simulink model "f_cd_reorder_one_interface"  (R2018a)
settings: Solver=VariableStepAuto  StartTime=0.0  StopTime=200000  RelTol=1e-3
libraries: xbsIndex_r4 x1754, casper_library_misc x12, xps_library x2, simulink x1
(part 2 of 9)

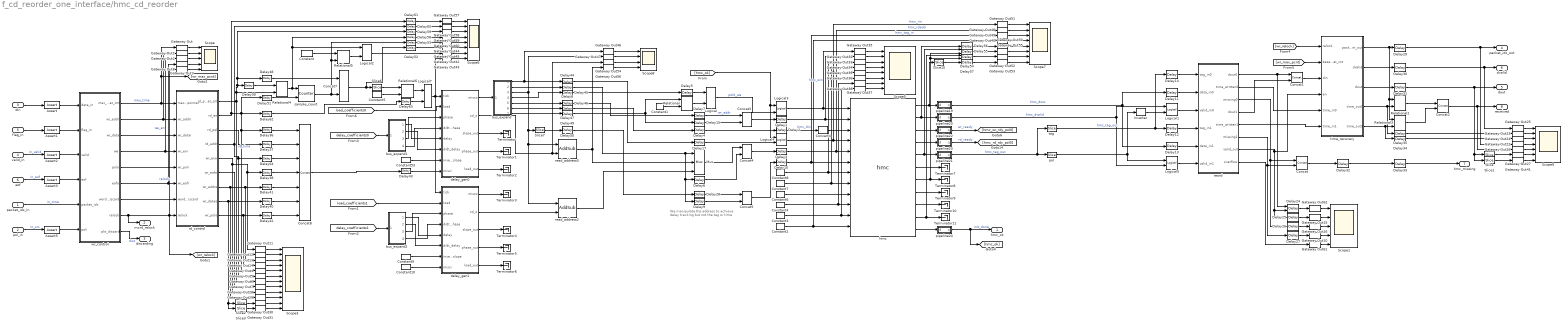
== system f_cd_reorder_one_interface/hmc_cd_reorder ==
  note: We manipulate the address to
      | achieve delay tracking but not the tag
      | or time
  packet_idx_in : Inport
  pol_in : Inport  Port=2
  din : Inport  Port=3
  valid_in : Inport  Port=4
  flag_in : Inport  Port=5
  eof : Inport  Port=6
  Assert : xbsIndex_r4/Assert  assert_type=on  type_source=Explicitly  gui_display_data_type=Fixed-point  arith_type=Unsigned  n_bits=n_bits_din  bin_pt=0  preci_type=Single  exp_width=8  frac_width=24  assert_rate=off  rate_source=Explicitly  period=1  output_port=on  block_type=assert
  Assert1 : xbsIndex_r4/Assert  assert_type=on  type_source=Explicitly  gui_display_data_type=Fixed-point  arith_type=Unsigned  n_bits=n_bits_flag  bin_pt=0  preci_type=Single  exp_width=8  frac_width=24  assert_rate=off  rate_source=Explicitly  period=1  output_port=on  block_type=assert
  Assert2 : xbsIndex_r4/Assert  assert_type=on  type_source=Explicitly  gui_display_data_type=Boolean  arith_type=Boolean  n_bits=n_bits_flag  bin_pt=0  preci_type=Single  exp_width=8  frac_width=24  assert_rate=off  rate_source=Explicitly  period=1  output_port=on  block_type=assert
  Assert3 : xbsIndex_r4/Assert  assert_type=on  type_source=Explicitly  gui_display_data_type=Boolean  arith_type=Boolean  n_bits=n_bits_flag  bin_pt=0  preci_type=Single  exp_width=8  frac_width=24  assert_rate=off  rate_source=Explicitly  period=1  output_port=on  block_type=assert
  Assert5 : xbsIndex_r4/Assert  assert_type=on  type_source=Explicitly  gui_display_data_type=Fixed-point  arith_type=Unsigned  n_bits=1  bin_pt=0  preci_type=Single  exp_width=8  frac_width=24  assert_rate=off  rate_source=Explicitly  period=1  output_port=on  block_type=assert
  Concat{,1..5,7} (7 alike) : xbsIndex_r4/Concat  num_inputs=2  dbl_ovrd=off  block_type=concat
  Concat8 : xbsIndex_r4/Concat  num_inputs=7  dbl_ovrd=off  block_type=concat
  Constant : xbsIndex_r4/Constant  const=(packet_size-1)*samples_per_word*2  gui_display_data_type=Fixed-point  arith_type=Unsigned  n_bits=ceil(log2(packet_size*samples_per_word))+1  bin_pt=0  preci_type=Single  exp_width=8  frac_width=24  explicit_period=on  period=1  equ=P=C  opselect=C  inp2=PCIN>>17  opr=+  inp1=P  carry=CIN  dbl_ovrd=off  block_type=constant
  Constant1 : xbsIndex_r4/Constant  const=0  gui_display_data_type=Fixed-point  arith_type=Unsigned  n_bits=1  bin_pt=0  preci_type=Single  exp_width=8  frac_width=24  explicit_period=on  period=1  equ=P=C  opselect=C  inp2=PCIN>>17  opr=+  inp1=P  carry=CIN  dbl_ovrd=off  block_type=constant
  Constant10 : xbsIndex_r4/Constant  const=0  gui_display_data_type=Boolean  arith_type=Boolean  n_bits=1  bin_pt=0  preci_type=Single  exp_width=8  frac_width=24  explicit_period=on  period=1  equ=P=C  opselect=C  inp2=PCIN>>17  opr=+  inp1=P  carry=CIN  dbl_ovrd=off  block_type=constant
      settings: block_version=11.4
  Constant2 : xbsIndex_r4/Constant  const=0  gui_display_data_type=Fixed-point  arith_type=Unsigned  n_bits=9  bin_pt=0  preci_type=Single  exp_width=8  frac_width=24  explicit_period=on  period=1  equ=P=C  opselect=C  inp2=PCIN>>17  opr=+  inp1=P  carry=CIN  dbl_ovrd=off  block_type=constant
  Constant3 : xbsIndex_r4/Constant  const=0  gui_display_data_type=Fixed-point  arith_type=Unsigned  n_bits=n_bits_buffer_size  bin_pt=0  preci_type=Single  exp_width=8  frac_width=24  explicit_period=on  period=1  equ=P=C  opselect=C  inp2=PCIN>>17  opr=+  inp1=P  carry=CIN  dbl_ovrd=off  block_type=constant
  Constant4 : xbsIndex_r4/Constant  const=0  gui_display_data_type=Boolean  arith_type=Boolean  n_bits=n_bits_buffer_size  bin_pt=0  preci_type=Single  exp_width=8  frac_width=24  explicit_period=on  period=1  equ=P=C  opselect=C  inp2=PCIN>>17  opr=+  inp1=P  carry=CIN  dbl_ovrd=off  block_type=constant
  Constant5 : xbsIndex_r4/Constant  const=0  gui_display_data_type=Fixed-point  arith_type=Unsigned  n_bits=n_bits_fft+1  bin_pt=0  preci_type=Single  exp_width=8  frac_width=24  explicit_period=on  period=1  equ=P=C  opselect=C  inp2=PCIN>>17  opr=+  inp1=P  carry=CIN  dbl_ovrd=off  block_type=constant
  Constant53 : xbsIndex_r4/Constant  const=0  gui_display_data_type=Boolean  arith_type=Boolean  n_bits=1  bin_pt=0  preci_type=Single  exp_width=8  frac_width=24  explicit_period=on  period=1  equ=P=C  opselect=C  inp2=PCIN>>17  opr=+  inp1=P  carry=CIN  dbl_ovrd=off  block_type=constant
      settings: block_version=11.4
  Constant6 : xbsIndex_r4/Constant  const=0  gui_display_data_type=Fixed-point  arith_type=Unsigned  n_bits=256  bin_pt=0  preci_type=Single  exp_width=8  frac_width=24  explicit_period=on  period=1  equ=P=C  opselect=C  inp2=PCIN>>17  opr=+  inp1=P  carry=CIN  dbl_ovrd=off  block_type=constant
  Constant7 : xbsIndex_r4/Constant  const=0  gui_display_data_type=Fixed-point  arith_type=Unsigned  n_bits=n_bits_buffer_size  bin_pt=0  preci_type=Single  exp_width=8  frac_width=24  explicit_period=on  period=1  equ=P=C  opselect=C  inp2=PCIN>>17  opr=+  inp1=P  carry=CIN  dbl_ovrd=off  block_type=constant
  Constant8 : xbsIndex_r4/Constant  const=0  gui_display_data_type=Boolean  arith_type=Boolean  n_bits=n_bits_buffer_size  bin_pt=0  preci_type=Single  exp_width=8  frac_width=24  explicit_period=on  period=1  equ=P=C  opselect=C  inp2=PCIN>>17  opr=+  inp1=P  carry=CIN  dbl_ovrd=off  block_type=constant
  Constant9 : xbsIndex_r4/Constant  const=0  gui_display_data_type=Boolean  arith_type=Boolean  n_bits=1  bin_pt=0  preci_type=Single  exp_width=8  frac_width=24  explicit_period=on  period=1  equ=P=C  opselect=C  inp2=PCIN>>17  opr=+  inp1=P  carry=CIN  dbl_ovrd=off  block_type=constant
      settings: block_version=11.4
  Convert4 : xbsIndex_r4/Convert  gui_display_data_type=Fixed-point  arith_type=Unsigned  n_bits=256  bin_pt=0  float_type=Single  exp_bits=8  fraction_bits=24  quantization=Truncate  overflow=Wrap  en=off  latency=0  pipeline=off  dbl_ovrd=off  block_type=convert
  Delay{1..3,5,8,10..14,43..53,56..63} (29 alike) : xbsIndex_r4/Delay  rst=off  infoeditControl=Selection of Reset will increase slice count due to use of real FFs and instead of SRLs  en=off  latency=1  reg_retiming=on  dbl_ovrd=off  block_type=delay
      Delay1 settings: xl_area=[0, 0, 0, 0, 0, 0, 0]
      Delay10 settings: xl_area=[0, 0, 0, 0, 0, 0, 0]
      Delay2 settings: xl_area=[0, 0, 0, 0, 0, 0, 0]
      Delay3 settings: xl_area=[0, 0, 0, 0, 0, 0, 0]
      Delay44 settings: xl_area=[0, 0, 0, 0, 0, 0, 0]
      Delay45 settings: xl_area=[0, 0, 0, 0, 0, 0, 0]
      Delay46 settings: xl_area=[0, 0, 0, 0, 0, 0, 0]
      Delay47 settings: xl_area=[0, 0, 0, 0, 0, 0, 0]
      Delay49 settings: xl_area=[0, 0, 0, 0, 0, 0, 0]
      Delay5 settings: xl_area=[0, 0, 0, 0, 0, 0, 0]
      Delay50 settings: xl_area=[0, 0, 0, 0, 0, 0, 0]
      Delay56 settings: xl_area=[0, 0, 0, 0, 0, 0, 0]
      Delay57 settings: xl_area=[0, 0, 0, 0, 0, 0, 0]
      Delay8 settings: xl_area=[0, 0, 0, 0, 0, 0, 0]
  Delay{4,6..7,9,15,17,28} (7 alike) : xbsIndex_r4/Delay  rst=off  infoeditControl=Selection of Reset will increase slice count due to use of real FFs and instead of SRLs  en=off  latency=2  reg_retiming=on  dbl_ovrd=off  block_type=delay
      settings: xl_area=[0, 0, 0, 0, 0, 0, 0]
  Delay24 : xbsIndex_r4/Delay  rst=off  infoeditControl=Selection of Reset will increase slice count due to use of real FFs and instead of SRLs  en=on  latency=1  reg_retiming=off  dbl_ovrd=off  block_type=delay
  Delay{25..27,29..31,33..42,64} (17 alike) : xbsIndex_r4/Delay  rst=off  infoeditControl=Selection of Reset will increase slice count due to use of real FFs and instead of SRLs  en=off  latency=1  reg_retiming=off  dbl_ovrd=off  block_type=delay
  Delay32 : xbsIndex_r4/Delay  rst=off  infoeditControl=Selection of Reset will increase slice count due to use of real FFs and instead of SRLs  en=off  latency=2  reg_retiming=off  dbl_ovrd=off  block_type=delay
  Delay54 : xbsIndex_r4/Delay  rst=off  infoeditControl=Selection of Reset will increase slice count due to use of real FFs and instead of SRLs  en=on  latency=1  reg_retiming=on  dbl_ovrd=off  block_type=delay
      settings: xl_area=[0, 0, 0, 0, 0, 0, 0]
  Delay55 : xbsIndex_r4/Delay  rst=off  infoeditControl=Selection of Reset will increase slice count due to use of real FFs and instead of SRLs  en=on  latency=1  reg_retiming=on  dbl_ovrd=off  block_type=delay
      settings: xl_area=[0, 0, 0, 0, 0, 0, 0]
  Gateway Out{,1..8,11..14,28..40,42..60} (45 alike) : xbsIndex_r4/Gateway Out  inherit_from_input=off  hdl_port=off  rows=1  columns=1  UseAsDAC=off  DACChannel='1'  interface=None  automatic_assignment=on  address_offset=hex2dec('00')  intf_name=''  intf_description=''  timing_constraint=None  locs_specified=off  LOCs={}  io_standard={}  block_type=gatewayout
  Gateway Out{10,15..16,22..27,41,61..62} (12 alike) : xbsIndex_r4/Gateway Out  inherit_from_input=off  hdl_port=on  rows=1  columns=1  UseAsDAC=off  DACChannel='1'  interface=None  automatic_assignment=on  address_offset=hex2dec('00')  intf_name=''  intf_description=''  timing_constraint=None  locs_specified=off  LOCs={}  io_standard={}  block_type=gatewayout
  Inverter : xbsIndex_r4/Inverter  en=off  latency=0  dbl_ovrd=off  block_type=inv
  Logical{,1..5} (6 alike) : xbsIndex_r4/Logical  logical_function=AND  inputs=2  en=off  latency=1  precision=Full  arith_type=Unsigned  n_bits=16  bin_pt=0  align_bp=on  dbl_ovrd=off  block_type=logical
  Logical7 : xbsIndex_r4/Logical  logical_function=AND  inputs=2  en=off  latency=0  precision=Full  arith_type=Unsigned  n_bits=16  bin_pt=0  align_bp=on  dbl_ovrd=off  block_type=logical
  Mux : xbsIndex_r4/Mux  inputs=2  en=off  latency=2  precision=Full  arith_type=Unsigned  n_bits=16  bin_pt=14  quantization=Truncate  overflow=Wrap  dbl_ovrd=off  block_type=mux
  Relational{,2..3,6} (4 alike) : xbsIndex_r4/Relational  mode=a=b  op_type=Bool  en=off  latency=1  dbl_ovrd=off  block_type=relational
  Relational4 : xbsIndex_r4/Relational  mode=a!=b  op_type=Bool  en=off  latency=0  dbl_ovrd=off  block_type=relational
  Relational5 : xbsIndex_r4/Relational  mode=a!=b  op_type=Bool  en=off  latency=0  dbl_ovrd=off  block_type=relational
  Scope : Scope  NumInputPorts=5
  Scope1 : Scope  NumInputPorts=5
  Scope3 : Scope  NumInputPorts=12
  Scope5 : Scope  NumInputPorts=8
  Scope6 : Scope  NumInputPorts=8
  Scope7 : Scope  NumInputPorts=8
  Scope8 : Scope  NumInputPorts=4
  Scope9 : Scope  NumInputPorts=7
  Slice : xbsIndex_r4/Slice  nbits=80  boolean_output=off  mode=Upper Bit Location + Width  bit1=0  base1=MSB of Input  bit0=0  base0=LSB of Input  dbl_ovrd=off  block_type=slice
  Slice1 : xbsIndex_r4/Slice  nbits=80  boolean_output=off  mode=Lower Bit Location + Width  bit1=0  base1=MSB of Input  bit0=0  base0=LSB of Input  dbl_ovrd=off  block_type=slice
  Slice10 : xbsIndex_r4/Slice  nbits=39  boolean_output=off  mode=Lower Bit Location + Width  bit1=0  base1=MSB of Input  bit0=161  base0=LSB of Input  dbl_ovrd=off  block_type=slice
  Slice2 : xbsIndex_r4/Slice  nbits=80  boolean_output=off  mode=Lower Bit Location + Width  bit1=0  base1=MSB of Input  bit0=0  base0=LSB of Input  dbl_ovrd=off  block_type=slice
  Slice3 : xbsIndex_r4/Slice  nbits=80  boolean_output=off  mode=Lower Bit Location + Width  bit1=0  base1=MSB of Input  bit0=80  base0=LSB of Input  dbl_ovrd=off  block_type=slice
  Slice6 : xbsIndex_r4/Slice  nbits=n_bits_fft  boolean_output=off  mode=Lower Bit Location + Width  bit1=0  base1=MSB of Input  bit0=1  base0=LSB of Input  dbl_ovrd=off  block_type=slice
  Slice7 : xbsIndex_r4/Slice  nbits=8  boolean_output=off  mode=Lower Bit Location + Width  bit1=0  base1=MSB of Input  bit0=0  base0=LSB of Input  dbl_ovrd=off  block_type=slice
  Terminator{,1..11} (12 alike) : Terminator
  bus_expand : Subsystem  AncestorBlock=casper_library_flow_control/bus_expand  mask(bus_expand){mode=divisions of arbitrary size, outputNum=1, outputWidth=[1 1 n_bits_buffer_size-1 1 n_bits_buffer_size-1 n_bits_din+n_bits_timestamp+n_bits_flag 1], outputBinaryPt=[0 0 0 0 0 0 0], outputArithmeticType=[2 0 0 2 0 0 0], show_format=off, outputToWorkspace=off, variablePrefix=out, outputToModelAsWell=on}
      mask prompts: outputNum "Number of outputs:"; outputWidth "Output width [msb ... lsb]:"; outputBinaryPt "Output binary point position [msb ... lsb]:"; outputArithmeticType "Output arithmetic type (ufix=0, fix=1, bool=2) [msb ... lsb]:"; show_format "Print format string?"; outputToWorkspace "Output to workspace?"; variablePrefix "Variable name prefix:"; outputToModelAsWell "Output to model as well?"
      mask help:
      | Expands a 'bus' made using a bus_create or Xilinx
      | concat block.
      | The input will be divided into the specified number
      | of outputs with the specified arithmetic types.
      | Divisions are made from most significant bit.
      mask init:
      | bus_expand_init(gcb,...
      |     'mode', mode, ...
      |     'outputNum', outputNum, ...
      |     'outputWidth', outputWidth, ...
      |     'outputBinaryPt', outputBinaryPt, ...
      |     'outputArithmeticType', outputArithmeticType, ...
      |     'show_format', show_format, ...
      |     'outputToWorkspace', outputToWorkspace, ...
      |     'variablePrefix', variablePrefix, ...
      |     'outputToModelAsWell', outputToModelAsWell);
      settings: AttributesFormatString=7 outputs
      mask TypeOptions mode: divisions of equal size | divisions of arbitrary size
      mask Callback mode: bus_expand_callback();
      mask Callback outputWidth: bus_expand_callback();
      mask Callback outputToWorkspace: bus_expand_callback();
  bus_expand1 : Subsystem  mask(bus_expand){mode=divisions of arbitrary size, outputNum=1, outputWidth=[n_bits_max_delay+15 16 16 16], outputBinaryPt=[15 15 15 15], outputArithmeticType=[0 1 1 1], show_format=off, outputToWorkspace=off, variablePrefix=out, outputToModelAsWell=on}
      mask prompts: outputNum "Number of outputs:"; outputWidth "Output width [msb ... lsb]:"; outputBinaryPt "Output binary point position [msb ... lsb]:"; outputArithmeticType "Output arithmetic type (ufix=0, fix=1, bool=2) [msb ... lsb]:"; show_format "Print format string?"; outputToWorkspace "Output to workspace?"; variablePrefix "Variable name prefix:"; outputToModelAsWell "Output to model as well?"
      mask help:
      | Expands a 'bus' made using a bus_create or Xilinx
      | concat block.
      | The input will be divided into the specified number
      | of outputs with the specified arithmetic types.
      | Divisions are made from most significant bit.
      mask init: same as f_cd_reorder_one_interface/hmc_cd_reorder/bus_expand
      settings: AttributesFormatString=4 outputs
      mask TypeOptions mode: divisions of equal size | divisions of arbitrary size
      mask Callback mode: bus_expand_callback();
      mask Callback outputWidth: bus_expand_callback();
      mask Callback outputToWorkspace: bus_expand_callback();
  bus_expand2 : Subsystem  mask(bus_expand){mode=divisions of arbitrary size, outputNum=1, outputWidth=[n_bits_max_delay+15 16 16 16], outputBinaryPt=[15 15 15 15], outputArithmeticType=[0 1 1 1], show_format=off, outputToWorkspace=off, variablePrefix=out, outputToModelAsWell=on}
      mask prompts: outputNum "Number of outputs:"; outputWidth "Output width [msb ... lsb]:"; outputBinaryPt "Output binary point position [msb ... lsb]:"; outputArithmeticType "Output arithmetic type (ufix=0, fix=1, bool=2) [msb ... lsb]:"; show_format "Print format string?"; outputToWorkspace "Output to workspace?"; variablePrefix "Variable name prefix:"; outputToModelAsWell "Output to model as well?"
      mask help:
      | Expands a 'bus' made using a bus_create or Xilinx
      | concat block.
      | The input will be divided into the specified number
      | of outputs with the specified arithmetic types.
      | Divisions are made from most significant bit.
      mask init: same as f_cd_reorder_one_interface/hmc_cd_reorder/bus_expand
      settings: AttributesFormatString=4 outputs
      mask TypeOptions mode: divisions of equal size | divisions of arbitrary size
      mask Callback mode: bus_expand_callback();
      mask Callback outputWidth: bus_expand_callback();
      mask Callback outputToWorkspace: bus_expand_callback();
  delay_gen0 : Subsystem  mask{fft_len=n_bits_fft-1, add_latency=1, data_bits=10 * 8, n_bits_index=n_bits_fft-3, lookup_bits=11, cd_bits=n_bits_max_delay, delay_bits=n_bits_max_delay+15, delay_bin_pt=15, max_delay_rate=23, min_delay_rate=38, phase_bits=16, max_phase_rate=23, min_phase_rate=38}
      mask prompts: fft_len "Effective FFT size (2^?)"; add_latency "Add latency"; data_bits "Data width"; n_bits_index "Index width"; lookup_bits "DDS lookup table resolution (2*pi/2^?)"; cd_bits "Coarse delay range (2^? bits)"; delay_bits "Input delay resolution (bits)"; delay_bin_pt "Input delay binary point"; max_delay_rate "Max delay update rate (1/2^? samples/sample)"; min_delay_rate "Min (non-zero) delay update rate (1/2^? samples/sample)"; phase_bits "Input phase resolution (2*pi/2^? radians)"; max_phase_rate "Max phase update rate (1/2^? radians/sample)"; min_phase_rate "Min (non-zero) phase rate (1/2^? radians/sample)"
  delay_gen1 : Subsystem  mask{fft_len=n_bits_fft-1, add_latency=1, data_bits=10 * 8, n_bits_index=n_bits_fft-3, lookup_bits=11, cd_bits=n_bits_max_delay, delay_bits=n_bits_max_delay+15, delay_bin_pt=15, max_delay_rate=23, min_delay_rate=38, phase_bits=16, max_phase_rate=23, min_phase_rate=38}
      mask prompts: fft_len "Effective FFT size (2^?)"; add_latency "Add latency"; data_bits "Data width"; n_bits_index "Index width"; lookup_bits "DDS lookup table resolution (2*pi/2^?)"; cd_bits "Coarse delay range (2^? bits)"; delay_bits "Input delay resolution (bits)"; delay_bin_pt "Input delay binary point"; max_delay_rate "Max delay update rate (1/2^? samples/sample)"; min_delay_rate "Min (non-zero) delay update rate (1/2^? samples/sample)"; phase_bits "Input phase resolution (2*pi/2^? radians)"; max_phase_rate "Max phase update rate (1/2^? radians/sample)"; min_phase_rate "Min (non-zero) phase rate (1/2^? radians/sample)"
  hmc : xps_library/Memory/hmc  Tag=xps:hmc  mez=0  sim_depth=n_bits_buffer_size  sim_latency=10000  sim_rand=off
      settings: SourceProductName=CASPER XPS Blockset
  pipeline19 : Subsystem  Tag=cmac_delinked  mask(pipeline){csp_latency=2}
      mask prompts: csp_latency "Latency"
      mask help:
      | An explicitly laid-out delay line to avoid mapping to SRL16s
      | for use in pipelining to help achieve timing closure.
      mask init:
      | pipeline_init(gcb,'latency',csp_latency);
      settings: AttributesFormatString=Latency = %<latency>
      mask Display:
      | port_label('input', 1, 'd');
      | port_label('output', 1, 'q');
      | disp(['Z^-', num2str(csp_latency)]);
  pipeline20 : Subsystem  Tag=cmac_delinked  mask(pipeline){csp_latency=2}
      mask prompts: csp_latency "Latency"
      mask help:
      | An explicitly laid-out delay line to avoid mapping to SRL16s
      | for use in pipelining to help achieve timing closure.
      mask init:
      | pipeline_init(gcb,'latency',csp_latency);
      settings: AttributesFormatString=Latency = %<latency>
      mask Display:
      | port_label('input', 1, 'd');
      | port_label('output', 1, 'q');
      | disp(['Z^-', num2str(csp_latency)]);
  pipeline21 : Subsystem  Tag=cmac_delinked  mask(pipeline){csp_latency=2}
      mask prompts: csp_latency "Latency"
      mask help:
      | An explicitly laid-out delay line to avoid mapping to SRL16s
      | for use in pipelining to help achieve timing closure.
      mask init:
      | pipeline_init(gcb,'latency',csp_latency);
      settings: AttributesFormatString=Latency = %<latency>
      mask Display:
      | port_label('input', 1, 'd');
      | port_label('output', 1, 'q');
      | disp(['Z^-', num2str(csp_latency)]);
  pipeline22 : Subsystem  Tag=cmac_delinked  mask(pipeline){csp_latency=2}
      mask prompts: csp_latency "Latency"
      mask help:
      | An explicitly laid-out delay line to avoid mapping to SRL16s
      | for use in pipelining to help achieve timing closure.
      mask init:
      | pipeline_init(gcb,'latency',csp_latency);
      settings: AttributesFormatString=Latency = %<latency>
      mask Display:
      | port_label('input', 1, 'd');
      | port_label('output', 1, 'q');
      | disp(['Z^-', num2str(csp_latency)]);
  pipeline23 : Subsystem  Tag=cmac_delinked  mask(pipeline){csp_latency=2}
      mask prompts: csp_latency "Latency"
      mask help:
      | An explicitly laid-out delay line to avoid mapping to SRL16s
      | for use in pipelining to help achieve timing closure.
      mask init:
      | pipeline_init(gcb,'latency',csp_latency);
      settings: AttributesFormatString=Latency = %<latency>
      mask Display:
      | port_label('input', 1, 'd');
      | port_label('output', 1, 'q');
      | disp(['Z^-', num2str(csp_latency)]);
  pipeline24 : Subsystem  Tag=cmac_delinked  mask(pipeline){csp_latency=2}
      mask prompts: csp_latency "Latency"
      mask help:
      | An explicitly laid-out delay line to avoid mapping to SRL16s
      | for use in pipelining to help achieve timing closure.
      mask init:
      | pipeline_init(gcb,'latency',csp_latency);
      settings: AttributesFormatString=Latency = %<latency>
      mask Display:
      | port_label('input', 1, 'd');
      | port_label('output', 1, 'q');
      | disp(['Z^-', num2str(csp_latency)]);
  pol : xbsIndex_r4/Slice  nbits=1  boolean_output=on  mode=Lower Bit Location + Width  bit1=0  base1=MSB of Input  bit0=0  base0=LSB of Input  dbl_ovrd=off  block_type=slice
  rd_control : Subsystem
  read_address0 : xbsIndex_r4/AddSub  mode=Subtraction  use_carryin=off  use_carryout=off  en=off  latency=1  precision=User Defined  arith_type=Unsigned  n_bits=n_bits_buffer_size-1  bin_pt=0  quantization=Truncate  overflow=Wrap  use_behavioral_HDL=off  hw_selection=Fabric  pipelined=off  dbl_ovrd=off  block_type=addsub
  read_address2 : xbsIndex_r4/AddSub  mode=Subtraction  use_carryin=off  use_carryout=off  en=off  latency=1  precision=User Defined  arith_type=Unsigned  n_bits=n_bits_buffer_size-1  bin_pt=0  quantization=Truncate  overflow=Wrap  use_behavioral_HDL=off  hw_selection=Fabric  pipelined=off  dbl_ovrd=off  block_type=addsub
  reord : Subsystem  mask{n_bits_buffer=12, n_bits_tag=8, bram_latency=3, packet_size=log2(256), n_bits_timestamp=48-12, n_bits_buffer_size=15+1+1 - 5, n_bits_watchdog=n_bits_buffer_size-1}
      mask prompts: n_bits_buffer "buffer depth (2^?)"; n_bits_tag "tag length"; bram_latency "bram latency"; packet_size "packet_size (2^?)"; n_bits_timestamp "Timestamp bits (2^?)"; n_bits_buffer_size "Total buffer size"; n_bits_watchdog "Watchdog timeout period"
  sample_count : xbsIndex_r4/Counter  cnt_type=Free Running  cnt_to=Inf  operation=Up  start_count=0  cnt_by_val=samples_per_word  arith_type=Unsigned  n_bits=ceil(log2(samples_per_packet))+1  bin_pt=0  load_pin=off  rst=on  en=on  explicit_period=on  period=1  use_behavioral_HDL=off  implementation=Fabric  dbl_ovrd=off  block_type=counter
  tag : xbsIndex_r4/Slice  nbits=7  boolean_output=off  mode=Upper Bit Location + Width  bit1=0  base1=MSB of Input  bit0=0  base0=LSB of Input  dbl_ovrd=off  block_type=slice
  time_recovery : Subsystem
  wr_control : Subsystem
  hmc_ok : Outport
  mcnt_relock : Outport  Port=2
  discarding : Outport  Port=3
  packet_idx_out : Outport  Port=4
  dout : Outport  Port=5
  dvalid : Outport  Port=6
  hmc_missing : Outport  Port=7
  received : Outport  Port=8
  wires:
  wr_control/1(max_packet_cnt) -> [wr_max_pcnt], Gateway Out/1, rd_control/1(max_write_pointer)  "max_time"
  Constant1/1 -> Relational/2
  Relational/1 -> Logical/2
  Logical/1 -> Logical3/2  "pol0_we"
  Delay5/1 -> Logical/1
  wr_control/8(relock) -> Gateway Out8/1, [wr_relock], rd_control/8(relock), mcnt_relock/1  "relock"
  wr_control/9(pkt_discard) -> discarding/1  "disc"
  din/1 -> Assert/1
  flag_in/1 -> Assert1/1
  valid_in/1 -> Assert2/1  "in_valid"
  eof/1 -> Assert3/1  "in_eof"
  packet_idx_in/1 -> wr_control/5(packet_idx)  "in_time"
  pol_in/1 -> Assert5/1  "in_src"
  Assert/1 -> wr_control/1(data_in)
  Assert1/1 -> wr_control/2(flag_in)
  Assert2/1 -> wr_control/3(valid)
  Assert3/1 -> wr_control/4(eof)
  Assert5/1 -> wr_control/6(poli)
  pipeline24/1(q) -> [hmc_ok], hmc_ok/1  "init_done"
  hmc/9 -> Terminator10/1
  hmc/7 -> Terminator8/1, Delay55/2, Delay54/2
  hmc/3 -> pipeline22/1(d)
  Logical4/1 -> hmc/4, Gateway Out51/1, Gateway Out39/1  "hmc_rin"
  Constant8/1 -> hmc/7, Gateway Out33/1
  pipeline21/1(q) -> tag/1, pol/1  "hmc_tag_out"
  hmc/2 -> pipeline20/1(d), Delay56/1
  Delay10/1 -> Gateway Out49/1, hmc/6  "hmc_tag_in"
  hmc/8 -> Terminator9/1
  pipeline20/1(q) -> Logical5/2, Logical1/1  "hmc_dvalid"
  hmc/5 -> pipeline21/1(d), Delay55/1
  hmc/6 -> Terminator7/1
  pipeline22/1(q) -> [hmc_wr_rdy_pol0]  "wr_ready"
  Constant7/1 -> hmc/8, Gateway Out34/1
  hmc/1 -> pipeline19/1(d), Slice10/1
  Constant4/1 -> hmc/10, Gateway Out37/1
  Delay1/1 -> hmc/2, Gateway Out32/1
  Delay2/1 -> Convert4/1  "hmc_din"
  Logical3/1 -> hmc/1, Gateway Out35/1  "hmc_win"
  pipeline19/1(q) -> Delay13/1, Delay11/1  "hmc_dout"
  Delay4/1 -> Delay2/1
  [hmc_ok] -> Logical4/1, Logical3/1
  hmc/4 -> pipeline23/1(d)
  Constant6/1 -> hmc/9
  pipeline23/1(q) -> [hmc_rd_rdy_pol0]  "rd_ready"
  hmc/11 -> pipeline24/1(d)
  wr_control/2(wr_addr) -> Gateway Out1/1, rd_control/2(wr_addri)
  wr_control/3(wr_data) -> rd_control/3(wr_datai)
  wr_control/4(we) -> Gateway Out2/1, rd_control/4(wr_eni)  "we_en"
  wr_control/5(polo) -> rd_control/5(wr_poli)
  wr_control/6(eofo) -> Gateway Out3/1, rd_control/6(wr_eofi)
  rd_control/9(wr_polo) -> Gateway Out14/1, Delay42/1
  rd_control/5(wr_eno) -> Gateway Out28/1, Delay38/1, Gateway Out11/1
  rd_control/8(wr_datao) -> Slice3/1, Slice2/1, Delay40/1
  Delay15/1 -> Concat3/2
  Concat3/1 -> Delay1/1
  Delay7/1 -> Concat3/1  "wr_addr"
  rd_control/7(wr_addro) -> Gateway Out29/1, Delay41/1, Gateway Out13/1
  Delay17/1 -> Logical4/2
  Delay8/1 -> Delay9/1, Delay6/1, Mux/1
  Gateway Out/1 -> Scope/1
  Gateway Out1/1 -> Scope/2
  Gateway Out2/1 -> Scope/3
  Gateway Out3/1 -> Scope/4
  Gateway Out14/1 -> Scope3/4
  Gateway Out12/1 -> Scope3/2
  Gateway Out11/1 -> Scope3/1
  Gateway Out13/1 -> Scope3/3
  rd_control/6(wr_eofo) -> Gateway Out12/1, Gateway Out7/1
  rd_control/1(rd_packet_cnt) -> Gateway Out6/1, Delay59/1, Delay48/1, Delay39/1, Relational4/2  "rd_time"
  Gateway Out4/1 -> Scope3/5
  Gateway Out5/1 -> Scope3/6
  Gateway Out6/1 -> Scope3/7
  Gateway Out7/1 -> Scope3/8
  Gateway Out8/1 -> Scope/5
  Delay3/1 -> hmc/5, Gateway Out48/1, Gateway Out36/1  "hmc_rdadd"
  Constant3/1 -> hmc/11, Gateway Out38/1
  Gateway Out28/1 -> Scope3/9
  Gateway Out29/1 -> Scope3/10
  Gateway Out30/1 -> Scope3/11
  Gateway Out31/1 -> Scope3/12
  Slice2/1 -> Gateway Out30/1
  Slice3/1 -> Gateway Out31/1
  Gateway Out35/1 -> Scope5/1
  Gateway Out34/1 -> Scope5/4
  Gateway Out32/1 -> Scope5/2
  Gateway Out33/1 -> Scope5/3
  Gateway Out39/1 -> Scope5/5
  Gateway Out36/1 -> Scope5/6
  Gateway Out37/1 -> Scope5/7
  Gateway Out38/1 -> Scope5/8
  Convert4/1 -> hmc/3
  Gateway Out49/1 -> Scope7/3
  Gateway Out48/1 -> Scope7/2
  Gateway Out51/1 -> Scope7/1
  hmc/10 -> Terminator11/1, Delay54/1
  Slice10/1 -> Delay57/1
  Gateway Out50/1 -> Scope7/5
  Gateway Out55/1 -> Scope7/6
  Gateway Out52/1 -> Scope7/7
  Gateway Out53/1 -> Scope7/8
  Gateway Out40/1 -> Scope7/4
  bus_expand1/4(lsb_out1) -> delay_gen0/4(d/dt_phase)
  Constant53/1 -> delay_gen0/7(invert_slope)
  [load_coefficients0] -> delay_gen0/2(load)
  bus_expand1/2(out3) -> delay_gen0/6(d/dt_delay)
  bus_expand1/1(msb_out4) -> delay_gen0/5(delay)
  Concat8/1 -> Delay43/1
  bus_expand1/3(out2) -> delay_gen0/3(phase)
  Delay39/1 -> Relational4/1
  sample_count/1 -> Concat7/2, Delay53/1, Relational5/2
  Constant/1 -> Relational5/1
  Relational5/1 -> Logical2/2
  Delay48/1 -> Concat7/1
  Concat7/1 -> Slice6/1, Delay52/1
  Slice6/1 -> Relational6/1
  Constant5/1 -> Relational6/2
  [delay_coefficients0] -> bus_expand1/1(bus_in)
  delay_gen0/1(misco) -> bus_expand/1(bus_in)
  delay_gen0/3(slope_out) -> Terminator/1
  delay_gen0/4(phase_out) -> Terminator1/1
  delay_gen0/5(load_out) -> Terminator2/1
  delay_gen0/2(cd_o) -> Gateway Out54/1, read_address0/2
  Delay43/1 -> delay_gen0/8(misci)
  Delay36/1 -> Concat8/1
  Delay37/1 -> Concat8/2
  bus_expand/1(msb_out7) -> Delay44/1, Gateway Out46/1
  bus_expand/3(out5) -> Gateway Out47/1, read_address2/1, read_address0/1, Slice7/1
  bus_expand/4(out4) -> Delay45/1
  bus_expand/5(out3) -> Delay46/1
  bus_expand/7(lsb_out1) -> Delay49/1
  bus_expand/6(out2) -> Delay47/1
  read_address0/1 -> Mux/2, Gateway Out56/1
  Delay44/1 -> Delay17/1
  read_address2/1 -> Mux/3
  Delay45/1 -> Delay5/1
  Delay46/1 -> Delay7/1
  Delay47/1 -> Delay4/1
  Delay49/1 -> Relational/1, Delay15/1
  Slice7/1 -> Delay50/1
  Delay50/1 -> Delay28/1
  Gateway Out46/1 -> Scope8/1
  Gateway Out47/1 -> Scope8/2
  Gateway Out54/1 -> Scope8/3
  Gateway Out56/1 -> Scope8/4
  Gateway Out57/1 -> Scope6/1
  Gateway Out58/1 -> Scope6/2
  Gateway Out59/1 -> Scope6/3
  Logical2/1 -> Gateway Out42/1
  Delay52/1 -> Gateway Out45/1
  Delay53/1 -> Gateway Out44/1
  Relational4/1 -> Delay58/1, Logical2/1, sample_count/1
  rd_control/4(rd_addr) -> Delay64/1, Gateway Out5/1, Delay60/1
  rd_control/2(rd_en) -> Delay61/1, Gateway Out4/1, Delay36/1, Delay62/1, Delay51/1
  Gateway Out60/1 -> Scope6/4
  Gateway Out44/1 -> Scope6/5
  Gateway Out45/1 -> Scope6/6
  Gateway Out42/1 -> Scope6/7
  Gateway Out43/1 -> Scope6/8
  Delay58/1 -> Gateway Out60/1
  Delay59/1 -> Gateway Out59/1
  Delay60/1 -> Gateway Out58/1
  Delay61/1 -> Gateway Out57/1
  Logical7/1 -> delay_gen1/1(tick), Gateway Out43/1, delay_gen0/1(tick)
  Relational6/1 -> Logical7/1
  Delay62/1 -> Delay63/1
  Delay63/1 -> Logical7/2
  Delay51/1 -> sample_count/2
  Delay54/1 -> Gateway Out52/1
  Delay55/1 -> Gateway Out55/1
  Delay56/1 -> Gateway Out50/1
  Delay57/1 -> Gateway Out53/1
  Delay42/1 -> Concat8/7
  Delay40/1 -> Concat8/6
  Delay41/1 -> Concat8/5
  Delay38/1 -> Concat8/4
  Delay64/1 -> Concat8/3
  rd_control/3(rd_pol) -> Delay37/1
  bus_expand/2(out6) -> Delay8/1
  Delay6/1 -> Concat4/2
  Constant2/1 -> hmc/12, Gateway Out40/1
  [load_coefficients1] -> delay_gen1/2(load)
  [delay_coefficients1] -> bus_expand2/1(bus_in)
  bus_expand2/3(out2) -> delay_gen1/3(phase)
  bus_expand2/1(msb_out4) -> delay_gen1/5(delay)
  bus_expand2/2(out3) -> delay_gen1/6(d/dt_delay)
  bus_expand2/4(lsb_out1) -> delay_gen1/4(d/dt_phase)
  Constant9/1 -> delay_gen1/7(invert_slope)
  Constant10/1 -> delay_gen1/8(misci)
  delay_gen1/5(load_out) -> Terminator6/1
  delay_gen1/4(phase_out) -> Terminator5/1
  delay_gen1/3(slope_out) -> Terminator4/1
  delay_gen1/1(misco) -> Terminator3/1
  delay_gen1/2(cd_o) -> read_address2/2
  Mux/1 -> Concat4/1
  Concat4/1 -> Delay3/1
  Delay28/1 -> Concat5/1
  Delay9/1 -> Concat5/2
  Concat5/1 -> Delay10/1
  Gateway Out61/1 -> Scope1/5
  Delay24/1 -> Gateway Out62/1
  Delay29/1 -> packet_idx_out/1, Gateway Out22/1
  Slice/1 -> Gateway Out27/1
  time_recovery/5(time_out1) -> Delay34/1, Relational3/2
  Gateway Out22/1 -> Scope9/4
  reord/6(missing1) -> Delay27/1, Concat/2
  Gateway Out23/1 -> Scope9/2
  Delay25/1 -> Gateway Out15/1
  Delay26/1 -> Gateway Out16/1
  Concat1/1 -> time_recovery/3(din)
  Gateway Out24/1 -> Scope9/3
  Delay34/1 -> Gateway Out24/1
  reord/5(time_written1) -> time_recovery/6(time_in1)
  time_recovery/1(packet_cnt_out) -> Relational3/1, Relational2/1, Delay29/1
  time_recovery/3(dout) -> Delay31/1
  Relational3/1 -> Concat2/2
  time_recovery/2(dvalid) -> Delay30/1
  Gateway Out62/1 -> Scope1/1
  Gateway Out27/1 -> Scope9/6
  Concat/1 -> Delay32/1
  Logical5/1 -> reord/6(valid_in1)
  Gateway Out16/1 -> Scope1/3
  tag/1 -> Delay12/1, Delay14/1  "hmc_tag_out"
  Concat2/1 -> Gateway Out26/1, received/1
  reord/2(time_written0) -> time_recovery/5(time_in0)
  Gateway Out10/1 -> Scope1/4
  Delay33/1 -> hmc_missing/1
  Gateway Out41/1 -> Scope9/7
  reord/4(dout1) -> Concat1/2
  [wr_relock] -> time_recovery/1(relock)
  Gateway Out15/1 -> Scope1/2
  Logical1/1 -> reord/3(valid_in0)
  Delay31/1 -> Slice1/1, Slice/1, dout/1
  [wr_max_pcnt] -> time_recovery/2(base_packet_cnt)
  Delay27/1 -> Gateway Out10/1
  Gateway Out25/1 -> Scope9/1
  reord/3(missing0) -> Delay26/1, Concat/1
  time_recovery/4(time_out0) -> Delay35/1, Relational2/2
  Delay30/1 -> dvalid/1, Gateway Out25/1
  Slice1/1 -> Gateway Out41/1
  Delay35/1 -> Gateway Out23/1
  reord/7(valid_out) -> time_recovery/4(en), Delay25/1, Delay24/2
  Delay32/1 -> Delay33/1
  reord/8(overflow) -> Gateway Out61/1
  Relational2/1 -> Concat2/1
  reord/1(dout0) -> Delay24/1, Concat1/1
  Gateway Out26/1 -> Scope9/5
  Inverter/1 -> Logical1/2
  pol/1 -> Logical5/1, Inverter/1
  Delay13/1 -> reord/5(data_in1)
  Delay12/1 -> reord/4(tag_in1)
  Delay11/1 -> reord/2(data_in0)
  Delay14/1 -> reord/1(tag_in0)
  wr_control/7(word_discard) -> rd_control/7(word_discard)

== system f_cd_reorder_one_interface/munge2 ==
  din : Inport
  join : Subsystem  AncestorBlock=casper_library_flow_control/bus_create  mask(bus_create){inputNum=10}
      mask prompts: inputNum "Number of inputs:"
      mask init:
      | bus_create_init(gcb,...
      |     'inputNum', inputNum);
  reinterpret : xbsIndex_r4/Reinterpret  force_arith_type=on  arith_type=Unsigned  force_bin_pt=on  bin_pt=0  block_type=reinterpret
  reinterpret_out : xbsIndex_r4/Reinterpret  force_arith_type=on  arith_type=Unsigned  force_bin_pt=on  bin_pt=0  block_type=reinterpret
  split : Subsystem  AncestorBlock=casper_library_flow_control/bus_expand  mask(bus_expand){mode=divisions of arbitrary size, outputNum=1, outputWidth=[1 1 1 1 1 1 1 1 1 1], outputBinaryPt=[0 0 0 0 0 0 0 0 0 0], outputArithmeticType=[0 0 0 0 0 0 0 0 0 0], show_format=off, outputToWorkspace=off, variablePrefix=out, outputToModelAsWell=on}
      mask prompts: outputNum "Number of outputs:"; outputWidth "Output width [msb ... lsb]:"; outputBinaryPt "Output binary point position [msb ... lsb]:"; outputArithmeticType "Output arithmetic type (ufix=0, fix=1, bool=2) [msb ... lsb]:"; show_format "Print format string?"; outputToWorkspace "Output to workspace?"; variablePrefix "Variable name prefix:"; outputToModelAsWell "Output to model as well?"
      mask help:
      | Expands a 'bus' made using a bus_create or Xilinx
      | concat block.
      | The input will be divided into the specified number
      | of outputs with the specified arithmetic types.
      | Divisions are made from most significant bit.
      mask init: same as f_cd_reorder_one_interface/hmc_cd_reorder/bus_expand
      settings: AttributesFormatString=10 outputs
      mask TypeOptions mode: divisions of equal size | divisions of arbitrary size
      mask Callback mode: bus_expand_callback();
      mask Callback outputWidth: bus_expand_callback();
      mask Callback outputToWorkspace: bus_expand_callback();
  dout : Outport
  wires:
  reinterpret_out/1 -> dout/1
  din/1 -> reinterpret/1
  reinterpret/1 -> split/1(bus_in)
  join/1(bus_out) -> reinterpret_out/1
  split/1(msb_out10) -> join/1(in1)
  split/2(out9) -> join/2(in2)
  split/3(out8) -> join/3(in3)
  split/4(out7) -> join/4(in4)
  split/5(out6) -> join/5(in5)
  split/6(out5) -> join/6(in6)
  split/8(out3) -> join/7(in7)
  split/7(out4) -> join/8(in8)
  split/9(out2) -> join/9(in9)
  split/10(lsb_out1) -> join/10(in10)

== system f_cd_reorder_one_interface/tvg ==
  tvg_select : Inport
  en : Inport  Port=2
  din : Inport  Port=3
  timei : Inport  Port=4
  poli : Inport  Port=5
  eofi : Inport  Port=6
  Concat : xbsIndex_r4/Concat  num_inputs=5  dbl_ovrd=off  block_type=concat
  Constant : xbsIndex_r4/Constant  const=4  gui_display_data_type=Fixed-point  arith_type=Unsigned  n_bits=3  bin_pt=0  preci_type=Single  exp_width=8  frac_width=24  explicit_period=on  period=1  equ=P=C  opselect=C  inp2=PCIN>>17  opr=+  inp1=P  carry=CIN  dbl_ovrd=off  block_type=constant
  Constant1 : xbsIndex_r4/Constant  const=0  gui_display_data_type=Fixed-point  arith_type=Unsigned  n_bits=2  bin_pt=0  preci_type=Single  exp_width=8  frac_width=24  explicit_period=on  period=1  equ=P=C  opselect=C  inp2=PCIN>>17  opr=+  inp1=P  carry=CIN  dbl_ovrd=off  block_type=constant
  Counter : xbsIndex_r4/Counter  cnt_type=Count Limited  cnt_to=4  operation=Up  start_count=0  cnt_by_val=1  arith_type=Unsigned  n_bits=3  bin_pt=0  load_pin=off  rst=on  en=on  explicit_period=on  period=1  use_behavioral_HDL=off  implementation=Fabric  dbl_ovrd=off  block_type=counter
  Counter1 : xbsIndex_r4/Counter  cnt_type=Free Running  cnt_to=Inf  operation=Up  start_count=0  cnt_by_val=1  arith_type=Unsigned  n_bits=8-3  bin_pt=0  load_pin=off  rst=on  en=on  explicit_period=on  period=1  use_behavioral_HDL=off  implementation=Fabric  dbl_ovrd=off  block_type=counter
  Delay{1..10,13..20,24} (19 alike) : xbsIndex_r4/Delay  rst=off  infoeditControl=Selection of Reset will increase slice count due to use of real FFs and instead of SRLs  en=off  latency=1  reg_retiming=on  dbl_ovrd=off  block_type=delay
  Logical : xbsIndex_r4/Logical  logical_function=AND  inputs=2  en=off  latency=1  precision=Full  arith_type=Unsigned  n_bits=16  bin_pt=0  align_bp=on  dbl_ovrd=off  block_type=logical
  Mux : xbsIndex_r4/Mux  inputs=2  en=off  latency=1  precision=Full  arith_type=Unsigned  n_bits=16  bin_pt=14  quantization=Truncate  overflow=Wrap  dbl_ovrd=off  block_type=mux
  Relational : xbsIndex_r4/Relational  mode=a=b  op_type=Bool  en=off  latency=0  dbl_ovrd=off  block_type=relational
  bus_constant : Subsystem  AncestorBlock=casper_library_bus/bus_constant  mask(bus_constant){values=[0:15], n_bits=[4], bin_pts=[0], types=[0]}
      mask prompts: n_bits "bit widths"; bin_pts "binary points"; types "data type"
      mask help: Combine constants into a bus
      mask init:
      | bus_constant_init(gcb, ...
      |     'values', values, ...
      |     'n_bits', n_bits, ...
      |     'bin_pts', bin_pts, ...
      |     'types', types);
  bus_convert : Subsystem  AncestorBlock=casper_library_bus/bus_convert  mask(bus_convert){n_bits_in=(48)*ones(1,16), bin_pt_in=0, cmplx=off, n_bits_out=80, bin_pt_out=0, quantization=0, overflow=0, csp_latency=0, of=off, misc=off}
      mask prompts: n_bits_in "input bit widths"; bin_pt_in "input binary points"; cmplx "input complex"; n_bits_out "output bit widths"; bin_pt_out "output binary points"; quantization "quantization strategy (Truncate=0, Round  (unbiased: +/- Inf)=1, Round (unbiased: Even Values)=2)"; overflow "overflow strategy (Wrap=0, Saturate=1, Flag as error=2)"; csp_latency "latency"; of "overflow indication"; misc "misc support"
      mask help: Convert components of busses
      mask init:
      | bus_convert_init(gcb, ...
      |     'n_bits_in', n_bits_in, ...
      |     'bin_pt_in', bin_pt_in, ...
      |     'cmplx', cmplx, ...
      |     'n_bits_out', n_bits_out, ...
      |     'bin_pt_out', bin_pt_out, ...
      |     'quantization', quantization, ...
      |     'overflow', overflow, ...
      |     'csp_latency', csp_latency, ...
      |     'misc', misc, ...
      |     'of', of);
  bus_mux : Subsystem  AncestorBlock=casper_library_bus/bus_mux  mask(bus_mux){n_inputs=1, n_bits=[256 256 256 256 256], cmplx=off, misc=off, mux_latency=1}
      mask prompts: n_inputs "number of inputs"; n_bits "input bit widths"; cmplx "complex data"; misc "misc support"; mux_latency "mux latency"
      mask help: Mux components of bus
      mask init:
      | bus_mux_init(gcb, ...
      |     'n_inputs', n_inputs, ...
      |     'n_bits', n_bits, ...
      |     'cmplx', cmplx, ...
      |     'misc', misc, ...
      |     'mux_latency', mux_latency);
  munge : Subsystem  AncestorBlock=casper_library_flow_control/munge  mask(munge){divisions=18, div_size=[2+(48-12)+(8-3) 4*ones(1,16) 1], order=reshape([zeros(1,16); [1:16]; 17*ones(1, 16)], 1, 48), arith_type_out=Unsigned, bin_pt_out=0}
      mask prompts: divisions "Number of divisions"; div_size "Division size (bits)"; order "Division packing order"; arith_type_out "Output arithmetic type"; bin_pt_out "Output binary point"
      mask help: Splits an input bus into the specified number of divisions and then recombines them in the order specified (most significant division = 0,least = number divisions-1)
      mask init:
      | munge_init(gcb, ...
      |     'divisions', divisions, ...
      |     'div_size', div_size, ...
      |     'order', order, ...
      |     'arith_type_out', arith_type_out, ...
      |     'bin_pt_out', bin_pt_out);
      settings: AttributesFormatString=|
      | split:[43 4 4 4 4 4 4 4 4 4 4 4 4 4 4 4 4 1]
      | join:[0 1 17 0 2 17 0 3 17 0 4 17 0 5 17 0 6 17 0 7 17 0 8 17 0 9 17 0 10 17 0 11 17 0 12 17 0 13 17 0 14 17 0 15 17 0 16 17]
      | Unsigned [768,0]
      mask TypeOptions arith_type_out: Unsigned | Signed  (2's comp) | Floating-point
  dvalid : Outport
  dout : Outport  Port=2
  timeo : Outport  Port=3
  polo : Outport  Port=4
  eofo : Outport  Port=5
  wires:
  eofi/1 -> Counter/1, Delay15/1, Delay24/1
  en/1 -> Counter/2, Logical/2, Delay16/1
  munge/1(dout) -> bus_convert/1(din)
  Counter/1 -> Relational/1, Delay14/1
  din/1 -> Delay18/1
  poli/1 -> Delay17/1
  tvg_select/1 -> Delay19/1
  Delay2/1 -> Mux/2
  bus_mux/1(out) -> Mux/3
  Delay3/1 -> Mux/1
  Delay1/1 -> Delay4/1
  Delay5/1 -> Delay6/1
  Delay4/1 -> polo/1
  Mux/1 -> dout/1
  Delay8/1 -> Delay7/1
  Delay7/1 -> eofo/1
  Delay9/1 -> timeo/1
  Delay10/1 -> Delay9/1
  Concat/1 -> munge/1(din)
  timei/1 -> Delay13/1, Delay20/1
  bus_convert/1(dout) -> bus_mux/2(d0)
  Constant/1 -> Relational/2
  Relational/1 -> Logical/1
  Logical/1 -> Counter1/2
  Delay14/1 -> bus_mux/1(sel)
  Delay15/1 -> Delay8/1
  Delay16/1 -> Delay5/1
  Delay17/1 -> Concat/5, Delay1/1
  Delay18/1 -> Delay2/1
  Delay19/1 -> Delay3/1
  Delay20/1 -> Delay10/1
  Delay6/1 -> dvalid/1
  Delay24/1 -> Counter1/1
  bus_constant/1(dout) -> Concat/4
  Constant1/1 -> Concat/1
  Delay13/1 -> Concat/2
  Counter1/1 -> Concat/3

== system f_cd_reorder_one_interface/data_width_convert/bus_mux ==
  sel : Inport
  d0 : Inport  Port=2
  d_bussify : Subsystem  AncestorBlock=casper_library_flow_control/bus_create  mask(bus_create){inputNum=1}
      mask prompts: inputNum "Number of inputs:"
      mask init:
      | bus_create_init(gcb,...
      |     'inputNum', inputNum);
  expand0 : Subsystem  AncestorBlock=casper_library_flow_control/bus_expand  mask(bus_expand){mode=divisions of arbitrary size, outputNum=1, outputWidth=[160 160 160 160 160 160 160 160], outputBinaryPt=[0  0  0  0  0  0  0  0], outputArithmeticType=[0  0  0  0  0  0  0  0], show_format=on, outputToWorkspace=off, variablePrefix=, outputToModelAsWell=on}
      mask prompts: outputNum "Number of outputs:"; outputWidth "Output width [msb ... lsb]:"; outputBinaryPt "Output binary point position [msb ... lsb]:"; outputArithmeticType "Output arithmetic type (ufix=0, fix=1, bool=2) [msb ... lsb]:"; show_format "Print format string?"; outputToWorkspace "Output to workspace?"; variablePrefix "Variable name prefix:"; outputToModelAsWell "Output to model as well?"
      mask help:
      | Expands a 'bus' made using a bus_create or Xilinx
      | concat block.
      | The input will be divided into the specified number
      | of outputs with the specified arithmetic types.
      | Divisions are made from most significant bit.
      mask init: same as f_cd_reorder_one_interface/hmc_cd_reorder/bus_expand
      settings: AttributesFormatString=8 outputs: uf160.0,uf160.0,uf160.0,uf160.0,uf160.0,uf160.0,uf160.0,uf160.0,
      mask TypeOptions mode: divisions of equal size | divisions of arbitrary size
      mask Callback mode: bus_expand_callback();
      mask Callback outputWidth: bus_expand_callback();
      mask Callback outputToWorkspace: bus_expand_callback();
  mux0 : xbsIndex_r4/Mux  inputs=8  en=off  latency=3  precision=Full  arith_type=Unsigned  n_bits=16  bin_pt=14  quantization=Truncate  overflow=Wrap  dbl_ovrd=off  block_type=mux
  sel_expand : Subsystem  AncestorBlock=casper_library_flow_control/bus_expand  mask(bus_expand){mode=divisions of equal size, outputNum=1, outputWidth=3, outputBinaryPt=0, outputArithmeticType=0, show_format=on, outputToWorkspace=off, variablePrefix=, outputToModelAsWell=on}
      mask prompts: outputNum "Number of outputs:"; outputWidth "Output width:"; outputBinaryPt "Output binary point position:"; outputArithmeticType "Output arithmetic type (ufix=0, fix=1, bool=2):"; show_format "Print format string?"; outputToWorkspace "Output to workspace?"; variablePrefix "Variable name prefix:"; outputToModelAsWell "Output to model as well?"
      mask help:
      | Expands a 'bus' made using a bus_create or Xilinx
      | concat block.
      | The input will be divided into the specified number
      | of outputs with the specified arithmetic types.
      | Divisions are made from most significant bit.
      mask init: same as f_cd_reorder_one_interface/hmc_cd_reorder/bus_expand
      settings: AttributesFormatString=1 outputs: uf3.0,
      mask TypeOptions mode: divisions of equal size | divisions of arbitrary size
      mask Callback mode: bus_expand_callback();
      mask Callback outputWidth: bus_expand_callback();
      mask Callback outputToWorkspace: bus_expand_callback();
  out : Outport
  wires:
  sel/1 -> sel_expand/1(bus_in)
  d0/1 -> expand0/1(bus_in)
  sel_expand/1(msb_lsb_out1) -> mux0/1
  expand0/1(msb_out8) -> mux0/2
  expand0/2(out7) -> mux0/3
  expand0/3(out6) -> mux0/4
  expand0/4(out5) -> mux0/5
  expand0/5(out4) -> mux0/6
  expand0/6(out3) -> mux0/7
  expand0/7(out2) -> mux0/8
  expand0/8(lsb_out1) -> mux0/9
  mux0/1 -> d_bussify/1(in1)
  d_bussify/1(bus_out) -> out/1

== system f_cd_reorder_one_interface/data_width_convert/edge_detect ==
  in : Inport
  Delay : xbsIndex_r4/Delay  rst=off  infoeditControl=Selection of Reset will increase slice count due to use of real FFs and instead of SRLs  en=off  latency=1  reg_retiming=off  dbl_ovrd=off  block_type=delay
      settings: xl_area=[0, 0, 0, 0, 0, 0, 0]
  Inverter : xbsIndex_r4/Inverter  en=off  latency=0  dbl_ovrd=off  block_type=inv
      settings: xl_area=[0, 0, 0, 0, 0, 0, 0]
  edge_op : xbsIndex_r4/Logical  logical_function=AND  inputs=2  en=off  latency=0  precision=Full  arith_type=Unsigned  n_bits=8  bin_pt=2  align_bp=on  dbl_ovrd=off  block_type=logical
      settings: xl_area=[0, 0, 0, 0, 0, 0, 0]
  out : Outport
  wires:
  Inverter/1 -> edge_op/1
  edge_op/1 -> out/1
  in/1 -> Inverter/1, Delay/1
  Delay/1 -> edge_op/2
